simulink model "lift_hierarchy"  (R2020b)
settings: Solver=VariableStepAuto  StartTime=0.0  StopTime=10.0  RelTol=1e-3
settings Model: Creator=DELL  LastModifiedBy=DELL

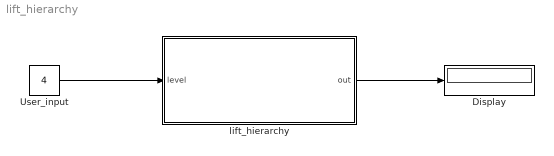
== system lift_hierarchy ==
  Display : Display
  User_input : Constant  Value=4
  lift_hierarchy : Stateflow chart  TreatAsAtomicUnit=on
  wires:
  User_input/1 -> lift_hierarchy/1(level)
  lift_hierarchy/1(out) -> Display/1

== stateflow chart lift_hierarchy/lift_hierarchy ==
  state Run_state
    state stop
      out=curr_st;
    state up
      entry:
      curr_st=curr_st+1;
      out=curr_st;
    state down
      entry:
      curr_st=curr_st-1;
      out=curr_st;
    (default) -> stop
    stop -> stop [order 1] : [level==curr_st]
    stop -> up [order 2] : [curr_st<level]
    stop -> down [order 3] : [curr_st>level]
    up -> stop [order 1] : [curr_st==level]
    down -> stop : [curr_st==level]
    up -> up [order 2] : [curr_st<level]
  state wait
    entry:
    cnt=0;
    du:
    cnt=cnt+1;
  (default) -> Run_state : {curr_st=0;}
  (junction 23) -> stop [order 3]
  (junction 23) -> up [order 1] : [curr_st<level]
  (junction 23) -> down [order 2] : [curr_st>level]
  Run_state -> wait : [curr_st~=level]
  wait -> (junction 23) : [cnt==2]
  data: cnt local; curr_st local =0; level input; out output
